simulink model "nlmpc_control_project"  (R2024b)
settings: Solver=ode45  StartTime=0.0  StopTime=tot_time  MaxStep=0.1  RelTol=1e-3
values from neighbouring files (symbols this model uses):
  g = 9.81    [main.m]    (also in mpc_control.m)
  Ib = diag([1.2416, 1.2416, 2 * 1.2416])    [getQuadrotorDynamicsAndJacobian.m]    (also in linearized_model.m = diag([Ib1 Ib2 Ib3]); main.m = diag([1.2416 1.2416 2*1.2416]))
  lin_vel_0 = [0 0 0]    [planner_1.m]    (also in planner_2.m = dot_p_d(1:3,1)')
  mass = 1.2    [getQuadrotorDynamicsAndJacobian.m]    (also in main.m)
  pos_0 = waypoints(1,1:3)    [planner_1.m]    (also in planner_2.m = p_d(1:3,1)')
  Ts = 0.001    [main.m]
  u_T0 = 11.772    [main.m]
  w_bb_0 = [0 0 0]    [planner_1.m]    (also in planner_2.m)
undefined symbols (not defined in the file or in its folder): dspblkCoreblockFVToolHelper, gcbh
libraries: robotcorelib x1, mpclib x1, uavutilslib x1
settings Model: PacingRate=10  Creator=marcomaffeo  LastModifiedBy=marcomaffeo

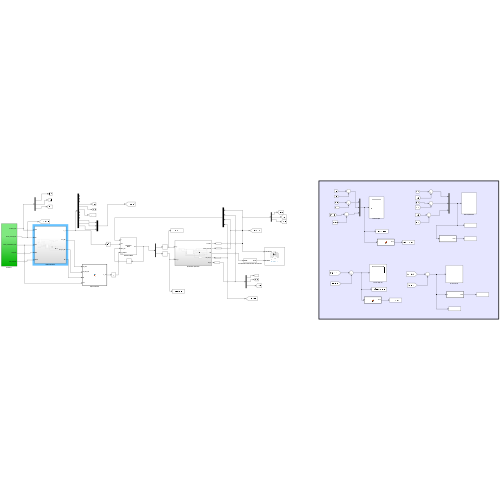
[thumbnail: Simulink's stored preview of the top-level diagram]
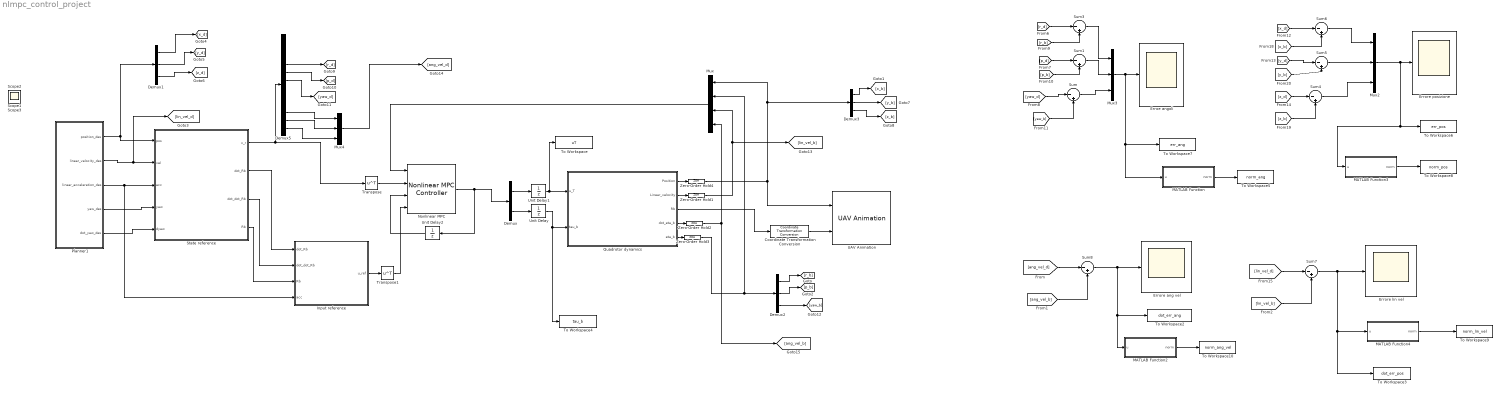
== system nlmpc_control_project ==
  Coordinate Transformation Conversion : robotcorelib/Coordinate Transformation Conversion  InputRepresentation=Rotation Matrix  InputEulerSequence=ZYX  ShowTrVecInputPort=on  OutputRepresentation=Quaternion  OutputEulerSequence=ZYX  ShowTrVecOutputPort=on  SimulateUsing=Interpreted execution
  Demux : Demux  Outputs=[1 3]
  Demux1 : Demux  Outputs=3
  Demux2 : Demux  Outputs=3
  Demux3 : Demux  Outputs=3
  Demux5 : Demux  Outputs=12
  Erroe angoli : Scope
  Errore ang vel : Scope
  Errore lin vel : Scope
  Errore posizione : Scope
  Input reference : MATLAB Function  TreatAsAtomicUnit=on
  MATLAB Function : MATLAB Function  TreatAsAtomicUnit=on
  MATLAB Function2 : MATLAB Function  TreatAsAtomicUnit=on
  MATLAB Function3 : MATLAB Function  TreatAsAtomicUnit=on
  MATLAB Function4 : MATLAB Function  TreatAsAtomicUnit=on
  Mux : Mux
  Mux2 : Mux  Inputs=3
  Mux3 : Mux  Inputs=3
  Mux4 : Mux  Inputs=3
  Nonlinear MPC : mpclib/Nonlinear MPC Controller  nlmpcobj=nlmpcobj  UseObjectTs=on  TsControl=-1  UseMEX=off  md_enabled=off  mvtarget_enabled=on  param_enabled=off  cost_enabled=off  mvseq_enabled=off  stateseq_enabled=off  ovseq_enabled=off  slack_enabled=off  status_enabled=off  ov_min=off  ov_max=off  mv_min=off  mv_max=off  mvrate_min=off  mvrate_max=off  state_min=off  state_max=off  ov_weight=off  mv_weight=off  mvrate_weight=off  ecr_weight=off  nlp_initialize=off
  Planner1 : Subsystem
  Quadrotor dynamics : Subsystem
  State reference : Subsystem
  Sum{,1,3..8} (8 alike) : Sum  Inputs=|-+
  To Workspace : ToWorkspace  VariableName=uT  SaveFormat=Structure With Time  SampleTime=Ts
  To Workspace10 : ToWorkspace  VariableName=norm_ang_vel  SaveFormat=Structure With Time  SampleTime=-1
  To Workspace2 : ToWorkspace  VariableName=dot_err_ang  SaveFormat=Structure With Time  SampleTime=Ts
  To Workspace3 : ToWorkspace  VariableName=dot_err_pos  SaveFormat=Structure With Time  SampleTime=-1
  To Workspace4 : ToWorkspace  VariableName=tau_b  SaveFormat=Structure With Time  SampleTime=Ts
  To Workspace5 : ToWorkspace  VariableName=norm_ang  SaveFormat=Structure With Time  SampleTime=-1
  To Workspace6 : ToWorkspace  VariableName=err_pos  SaveFormat=Structure With Time  SampleTime=Ts
  To Workspace7 : ToWorkspace  VariableName=err_ang  SaveFormat=Structure With Time  SampleTime=Ts
  To Workspace8 : ToWorkspace  VariableName=norm_pos  SaveFormat=Structure With Time  SampleTime=-1
  To Workspace9 : ToWorkspace  VariableName=norm_lin_vel  SaveFormat=Structure With Time  SampleTime=-1
  Transpose : Math  Operator=transpose
  Transpose1 : Math  Operator=transpose
  UAV Animation : uavutilslib/UAV Animation  NumUAV=1  DynamicUAVConfig=off  UAVType=Multirotor  UAVSize=1  UAVColor=[1 0.5 0]  UAVTrajectoryAlpha=1  InertialZDirection=Down  RotationFormat=Quaternion  DrawMarkers=off  SampleTime=0.01
  Unit Delay : UnitDelay  InitialCondition=[0 0 0]  SampleTime=Ts  HasFrameUpgradeWarning=on
  Unit Delay1 : UnitDelay  InitialCondition=u_T0  SampleTime=Ts  HasFrameUpgradeWarning=on
  Unit Delay2 : UnitDelay  InitialCondition=[u_T0 0 0 0]'  SampleTime=Ts  HasFrameUpgradeWarning=on
  Zero-Order Hold{1..4} (4 alike) : ZeroOrderHold  SampleTime=Ts
  Scope1 : Scope
  Scope2 : Scope
  Scope3 : Scope
  wires:
  Quadrotor dynamics/1(Position) -> Zero-Order Hold4/1
  Coordinate Transformation Conversion/1 -> UAV Animation/2
  Quadrotor dynamics/4(dot_eta_b) -> Zero-Order Hold2/1
  Quadrotor dynamics/3(Rb) -> Coordinate Transformation Conversion/1
  Demux/2 -> Unit Delay/1
  Planner1/1(position_des) -> State reference/1(pos), Demux1/1
  Planner1/2(linear_velocity_des) -> State reference/2(vel), [lin_vel_d]
  Planner1/3(linear_acceleration_des) -> State reference/3(acc), Input reference/4(acc)
  Planner1/4(yaw_des) -> State reference/4(yaw)
  Planner1/5(dot_yaw_des) -> State reference/5(dyaw)
  Unit Delay/1 -> To Workspace4/1, Quadrotor dynamics/2(tau_b)
  State reference/2(dot_Rb) -> Input reference/1(dot_Rb)
  State reference/3(dot_dot_Rb) -> Input reference/2(dot_dot_Rb)
  State reference/4(Rb) -> Input reference/3(Rb)
  Nonlinear MPC/1 -> Demux/1, Unit Delay2/1
  State reference/1(x_r) -> Demux5/1, Transpose/1
  Quadrotor dynamics/2(Linear_velocity) -> Zero-Order Hold1/1
  Transpose/1 -> Nonlinear MPC/2
  Input reference/1(u_ref) -> Transpose1/1
  Unit Delay2/1 -> Nonlinear MPC/3
  Demux3/1 -> [x_b]
  Demux3/2 -> [y_b]
  Demux3/3 -> [z_b]
  Transpose1/1 -> Nonlinear MPC/4
  Mux/1 -> Nonlinear MPC/1
  Zero-Order Hold4/1 -> Demux3/1, Mux/1, UAV Animation/1
  Zero-Order Hold1/1 -> Mux/3, [lin_vel_b]
  Zero-Order Hold2/1 -> Mux/4, [ang_vel_b]
  Demux2/1 -> [r_b]
  Demux2/2 -> [p_b]
  Unit Delay1/1 -> To Workspace/1, Quadrotor dynamics/1(u_T)
  Demux/1 -> Unit Delay1/1
  Demux1/1 -> [x_d]
  Demux1/2 -> [y_d]
  Demux1/3 -> [z_d]
  Demux2/3 -> [yaw_b]
  Demux5/4 -> [r_d]
  Demux5/5 -> [p_d]
  Demux5/6 -> [yaw_d]
  Demux5/10 -> Mux4/1
  Demux5/11 -> Mux4/2
  Demux5/12 -> Mux4/3
  Mux4/1 -> [ang_vel_d]
  Sum6/1 -> Mux2/1
  [x_d] -> Sum6/1
  [x_b] -> Sum6/2
  [y_d] -> Sum5/1
  [z_b] -> Sum4/2
  [ang_vel_d] -> Sum8/1
  MATLAB Function/1(norm) -> To Workspace5/1
  [yaw_b] -> Sum/2
  [z_d] -> Sum4/1
  MATLAB Function3/1(norm) -> To Workspace8/1
  MATLAB Function4/1(norm) -> To Workspace9/1
  Sum1/1 -> Mux3/2
  [lin_vel_d] -> Sum7/1
  [r_d] -> Sum3/1
  Sum5/1 -> Mux2/2
  [yaw_d] -> Sum/1
  [p_d] -> Sum1/1
  Sum/1 -> Mux3/3
  [p_b] -> Sum1/2
  Sum4/1 -> Mux2/3
  [lin_vel_b] -> Sum7/2
  [r_b] -> Sum3/2
  Mux3/1 -> Erroe angoli/1, To Workspace7/1, MATLAB Function/1(u)
  Mux2/1 -> MATLAB Function3/1(u), To Workspace6/1, Errore posizione/1
  Sum3/1 -> Mux3/1
  [ang_vel_b] -> Sum8/2
  Sum7/1 -> Errore lin vel/1, MATLAB Function4/1(u), To Workspace3/1
  [y_b] -> Sum5/2
  MATLAB Function2/1(norm) -> To Workspace10/1
  Sum8/1 -> Errore ang vel/1, MATLAB Function2/1(u), To Workspace2/1
  Quadrotor dynamics/5(eta_b) -> Zero-Order Hold3/1
  Zero-Order Hold3/1 -> Mux/2, Demux2/1

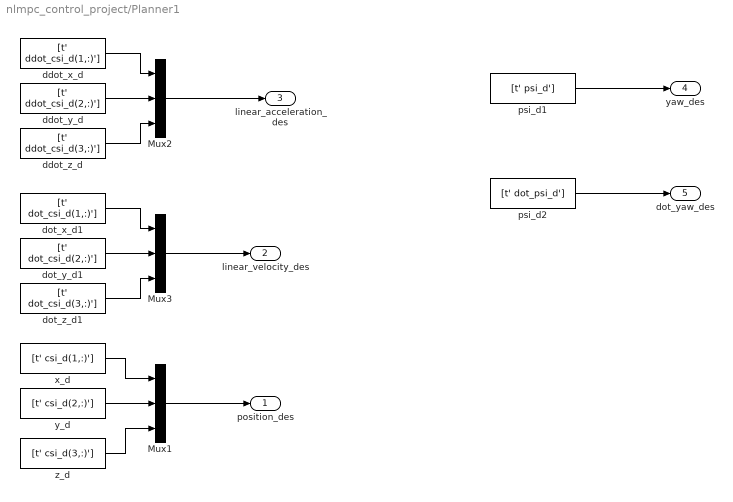
== system nlmpc_control_project/Planner1 ==
  Mux1 : Mux  Inputs=3
  Mux2 : Mux  Inputs=3
  Mux3 : Mux  Inputs=3
  ddot_x_d : FromWorkspace  VariableName=[t' ddot_csi_d(1,:)']  SampleTime=Ts
  ddot_y_d : FromWorkspace  VariableName=[t' ddot_csi_d(2,:)']  SampleTime=Ts
  ddot_z_d : FromWorkspace  VariableName=[t' ddot_csi_d(3,:)']  SampleTime=Ts
  dot_x_d1 : FromWorkspace  VariableName=[t' dot_csi_d(1,:)']  SampleTime=Ts
  dot_y_d1 : FromWorkspace  VariableName=[t' dot_csi_d(2,:)']  SampleTime=Ts
  dot_z_d1 : FromWorkspace  VariableName=[t' dot_csi_d(3,:)']  SampleTime=Ts
  psi_d1 : FromWorkspace  VariableName=[t' psi_d']  SampleTime=Ts
  psi_d2 : FromWorkspace  VariableName=[t' dot_psi_d']  SampleTime=Ts
  x_d : FromWorkspace  VariableName=[t' csi_d(1,:)']  SampleTime=Ts
  y_d : FromWorkspace  VariableName=[t' csi_d(2,:)']  SampleTime=Ts
  z_d : FromWorkspace  VariableName=[t' csi_d(3,:)']  SampleTime=Ts
  position_des : Outport
  linear_velocity_des : Outport  Port=2
  linear_acceleration_des : Outport  Port=3
  yaw_des : Outport  Port=4
  dot_yaw_des : Outport  Port=5
  wires:
  z_d/1 -> Mux1/3
  y_d/1 -> Mux1/2
  dot_z_d1/1 -> Mux3/3
  Mux1/1 -> position_des/1
  Mux3/1 -> linear_velocity_des/1
  ddot_z_d/1 -> Mux2/3
  ddot_x_d/1 -> Mux2/1
  dot_y_d1/1 -> Mux3/2
  x_d/1 -> Mux1/1
  dot_x_d1/1 -> Mux3/1
  ddot_y_d/1 -> Mux2/2
  Mux2/1 -> linear_acceleration_des/1
  psi_d1/1 -> yaw_des/1
  psi_d2/1 -> dot_yaw_des/1

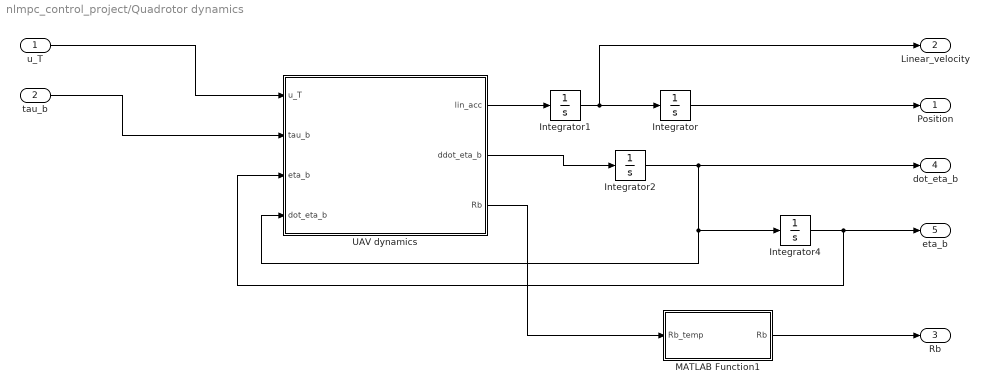
== system nlmpc_control_project/Quadrotor dynamics ==
  u_T : Inport
  tau_b : Inport  Port=2
  Integrator : Integrator  InitialCondition=pos_0
  Integrator1 : Integrator  InitialCondition=lin_vel_0
  Integrator2 : Integrator  InitialCondition=w_bb_0
  Integrator4 : Integrator  InitialCondition=[0 0 0]
  MATLAB Function1 : MATLAB Function  TreatAsAtomicUnit=on
  UAV dynamics : MATLAB Function  TreatAsAtomicUnit=on
  Position : Outport
  Linear_velocity : Outport  Port=2
  Rb : Outport  Port=3
  dot_eta_b : Outport  Port=4
  eta_b : Outport  Port=5
  wires:
  tau_b/1 -> UAV dynamics/2(tau_b)
  Integrator/1 -> Position/1
  UAV dynamics/1(lin_acc) -> Integrator1/1
  u_T/1 -> UAV dynamics/1(u_T)
  Integrator1/1 -> Linear_velocity/1, Integrator/1
  Integrator2/1 -> UAV dynamics/4(dot_eta_b), Integrator4/1, dot_eta_b/1
  Integrator4/1 -> UAV dynamics/3(eta_b), eta_b/1
  MATLAB Function1/1(Rb) -> Rb/1
  UAV dynamics/2(ddot_eta_b) -> Integrator2/1
  UAV dynamics/3(Rb) -> MATLAB Function1/1(Rb_temp)

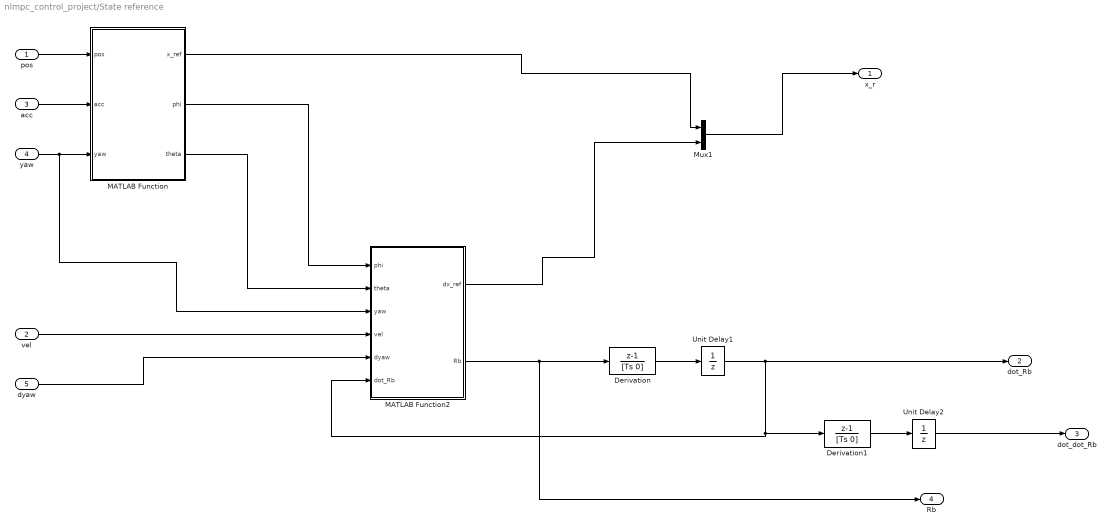
== system nlmpc_control_project/State reference ==
  pos : Inport
  vel : Inport  Port=2
  acc : Inport  Port=3
  yaw : Inport  Port=4
  dyaw : Inport  Port=5
  Derivation : DiscreteTransferFcn  LoadFcn=dspblkCoreblockFVToolHelper(gcbh,'load');  Numerator=[1 -1]  Denominator=[Ts 0]  InitialStates=[1 0 0;0 1 0;0 0 1]  SampleTime=Ts
      settings: CopyFcn=dspblkCoreblockFVToolHelper(gcbh,'copy');  DeleteFcn=dspblkCoreblockFVToolHelper(gcbh,'close');  ModelCloseFcn=dspblkCoreblockFVToolHelper(gcbh,'close');  PreSaveFcn=dspblkCoreblockFVToolHelper(gcbh,'presave');  PostSaveFcn=dspblkCoreblockFVToolHelper(gcbh,'postsave');  CloseFcn=dspblkCoreblockFVToolHelper(gcbh,'close');
  Derivation1 : DiscreteTransferFcn  LoadFcn=dspblkCoreblockFVToolHelper(gcbh,'load');  Numerator=[1 -1]  Denominator=[Ts 0]  InitialStates=[1 0 0;0 1 0;0 0 1]  SampleTime=Ts
      settings: CopyFcn=dspblkCoreblockFVToolHelper(gcbh,'copy');  DeleteFcn=dspblkCoreblockFVToolHelper(gcbh,'close');  ModelCloseFcn=dspblkCoreblockFVToolHelper(gcbh,'close');  PreSaveFcn=dspblkCoreblockFVToolHelper(gcbh,'presave');  PostSaveFcn=dspblkCoreblockFVToolHelper(gcbh,'postsave');  CloseFcn=dspblkCoreblockFVToolHelper(gcbh,'close');
  MATLAB Function : MATLAB Function  TreatAsAtomicUnit=on
  MATLAB Function2 : MATLAB Function  TreatAsAtomicUnit=on
  Mux1 : Mux  Inputs=2
  Unit Delay1 : UnitDelay  InitialCondition=eye(3)  SampleTime=Ts
  Unit Delay2 : UnitDelay  InitialCondition=eye(3)  SampleTime=Ts
  x_r : Outport
  dot_Rb : Outport  Port=2
  dot_dot_Rb : Outport  Port=3
  Rb : Outport  Port=4
  wires:
  pos/1 -> MATLAB Function/1(pos)
  acc/1 -> MATLAB Function/2(acc)
  dyaw/1 -> MATLAB Function2/5(dyaw)
  vel/1 -> MATLAB Function2/4(vel)
  yaw/1 -> MATLAB Function/3(yaw), MATLAB Function2/3(yaw)
  MATLAB Function/2(phi) -> MATLAB Function2/1(phi)
  MATLAB Function/3(theta) -> MATLAB Function2/2(theta)
  MATLAB Function2/1(dx_ref) -> Mux1/2
  Derivation/1 -> Unit Delay1/1
  Unit Delay1/1 -> dot_Rb/1, MATLAB Function2/6(dot_Rb), Derivation1/1
  Derivation1/1 -> Unit Delay2/1
  Unit Delay2/1 -> dot_dot_Rb/1
  MATLAB Function2/2(Rb) -> Derivation/1, Rb/1
  MATLAB Function/1(x_ref) -> Mux1/1
  Mux1/1 -> x_r/1

== matlab function nlmpc_control_project/MATLAB Function4 ==
  data: u input; norm output
function norm = fcn(u)

norm = sqrt(u(1)^2+u(2)^2+u(3)^2);

== matlab function nlmpc_control_project/State reference/MATLAB Function ==
  data: pos input; x_ref output; acc input; yaw input; g parameter; phi output; theta output
function [x_ref,phi,theta] = fcn(pos, acc, yaw, g)


x = pos(1); y = pos(2); z = pos(3);
ddx = acc(1); ddy = acc(2); ddz = -acc(3);


beta_a = -ddx * sin(yaw) + ddy * cos(yaw);
beta_c = -ddx * cos(yaw) + ddy * sin(yaw);
beta_d = -ddz + g;
beta_b = sqrt(beta_c^2 + beta_d^2);


phi = atan2(beta_a, beta_b);
theta = atan2(beta_c, beta_d);


x_ref = [x; y; z; phi; theta; yaw];
end

== matlab function nlmpc_control_project/Quadrotor dynamics/UAV dynamics ==
  data: u_T input size=1; tau_b input size=3; lin_acc output size=3; ddot_eta_b output size=3; eta_b input size=3; dot_eta_b input size=3; Rb output size=[3,3]; Ib parameter; mass parameter
function [lin_acc, ddot_eta_b,Rb] = fcn(u_T,tau_b,eta_b,dot_eta_b, Ib, mass)

%matrix definition
Q=[1              0                        -sin(eta_b(2));
   0        cos(eta_b(1))     cos(eta_b(2))*sin(eta_b(1));
   0       -sin(eta_b(1))    cos(eta_b(1))*cos(eta_b(2))];

Q_dot=[0             0                                                                          -cos(eta_b(2))*dot_eta_b(2);
       0 -sin(eta_b(1))*dot_eta_b(1)     -sin(eta_b(2))*sin(eta_b(1))*dot_eta_b(2)+cos(eta_b(2))*cos(eta_b(1))*dot_eta_b(1);
       0 -cos(eta_b(1))*dot_eta_b(1)     -sin(eta_b(2))*cos(eta_b(1))*dot_eta_b(2)-cos(eta_b(2))*sin(eta_b(1))*dot_eta_b(1)];


M=Q'*Ib*Q;

S = skew(Q*(dot_eta_b));

C = (Q'*S*Ib*Q)+ (Q'*Ib*Q_dot); 


Rb=[cos(eta_b(2))*cos(eta_b(3))   sin(eta_b(1))*sin(eta_b(2))*cos(eta_b(3))-cos(eta_b(1))*sin(eta_b(3))   cos(eta_b(1))*sin(eta_b(2))*cos(eta_b(3))+sin(eta_b(1))*sin(eta_b(3));
    cos(eta_b(2))*sin(eta_b(3))   sin(eta_b(1))*sin(eta_b(2))*sin(eta_b(3))+cos(eta_b(1))*cos(eta_b(3))   cos(eta_b(1))*sin(eta_b(2))*sin(eta_b(3))-sin(eta_b(1))*cos(eta_b(3));
        -sin(eta_b(2))              sin(eta_b(1))*cos(eta_b(2))                                           cos(eta_b(1))*cos(eta_b(2))];


%quadcopter dynamic model
lin_acc = 9.81*[0 0 1]'-(u_T/mass)*Rb*[0 0 1]';

ddot_eta_b = (inv(M))*((-C*dot_eta_b)+(Q'*tau_b));


end

function S = skew(v)
if(numel(v)~= 1)
S= [0 -v(3) v(2); 
    v(3) 0 -v(1);
    -v(2) v(1) 0];
else
S= zeros(3);
end
end

== matlab function nlmpc_control_project/Input reference ==
  data: dot_Rb input; dot_dot_Rb input; Rb input; acc input; u_ref output; g parameter; mass parameter; Ib parameter
function u_ref = fcn(dot_Rb,dot_dot_Rb,Rb,acc, g, mass, Ib)

% Calcolo thrust
u_T = mass * sqrt(acc(1)^2 + acc(2)^2 + (acc(3) - g)^2);


% Torques 
tau_b = Ib*wedge(dot_Rb'+Rb'*dot_dot_Rb)+((Rb'*dot_Rb*Ib)*(wedge(Rb'*dot_Rb)));

tau_phi = tau_b(1);
tau_theta = tau_b(2);
tau_psi = tau_b(3);

u_ref = [u_T; tau_phi; tau_theta; tau_psi];

end


function v = wedge(S)
v1 = S(3,2);
v2 = S(1,3);
v3 = S(2,1);
v = [v1 v2 v3]';
end

== matlab function nlmpc_control_project/Quadrotor dynamics/MATLAB Function1 ==
  data: Rb_temp input; Rb output
function Rb = fcn(Rb_temp)
    [U,S,V] = svd(Rb_temp);
    sigma = det(U*V');
    S_ = diag([1 1 sigma]);

    Rb = U*S_*V';
end

== matlab function nlmpc_control_project/State reference/MATLAB Function2 ==
  data: phi input; theta input; yaw input; dx_ref output; vel input; dyaw input; dot_Rb input; Rb output
function [dx_ref,Rb] = fcn(phi,theta,yaw,vel,dyaw,dot_Rb)

eta_b=[phi theta yaw]';

Rb=[cos(eta_b(2))*cos(eta_b(3))   sin(eta_b(1))*sin(eta_b(2))*cos(eta_b(3))-cos(eta_b(1))*sin(eta_b(3))   cos(eta_b(1))*sin(eta_b(2))*cos(eta_b(3))+sin(eta_b(1))*sin(eta_b(3));
    cos(eta_b(2))*sin(eta_b(3))   sin(eta_b(1))*sin(eta_b(2))*sin(eta_b(3))+cos(eta_b(1))*cos(eta_b(3))   cos(eta_b(1))*sin(eta_b(2))*sin(eta_b(3))-sin(eta_b(1))*cos(eta_b(3));
        -sin(eta_b(2))              sin(eta_b(1))*cos(eta_b(2))                                           cos(eta_b(1))*cos(eta_b(2))];


Q=[1              0                        -sin(eta_b(2));
   0        cos(eta_b(1))     cos(eta_b(2))*sin(eta_b(1));
   0       -sin(eta_b(1))    cos(eta_b(1))*cos(eta_b(2))];



dx = vel(1); dy = vel(2); dz = vel(3);


dot_eta_b=(inv(Q))*(wedge(Rb'*dot_Rb));

dphi = dot_eta_b(1);
dtheta = dot_eta_b(2);



dx_ref = [dx; dy; dz; dphi; dtheta; dyaw];


end

function v = wedge(S)
v1 = S(3,2);
v2 = S(1,3);
v3 = S(2,1);
v = [v1 v2 v3]';
end

== matlab function nlmpc_control_project/MATLAB Function ==
  data: u input; norm output
function norm = fcn(u)

norm = sqrt(u(1)^2+u(2)^2+u(3)^2);

== matlab function nlmpc_control_project/MATLAB Function2 ==
  data: u input; norm output
function norm = fcn(u)

norm = sqrt(u(1)^2+u(2)^2+u(3)^2);

== matlab function nlmpc_control_project/MATLAB Function3 ==
  data: u input; norm output
function norm = fcn(u)

norm = sqrt(u(1)^2+u(2)^2+u(3)^2);
